simulink model "Inverter_block_for_test"  (R2022b)
settings: Solver=VariableStepAuto  StartTime=0.0  StopTime=10.0  RelTol=1e-3
libraries: rtican x2
settings Model: Creator=tiszu  LastModifiedBy=tiszu

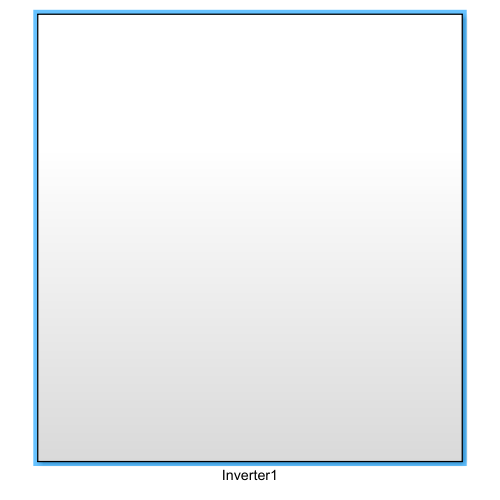
[thumbnail: Simulink's stored preview of the top-level diagram]
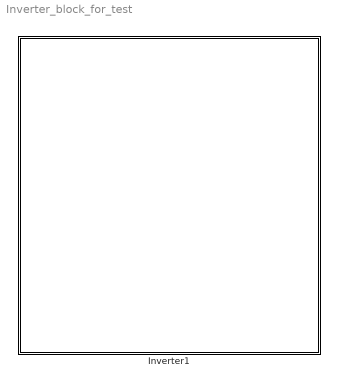
== system Inverter_block_for_test ==
  Inverter1 : Subsystem

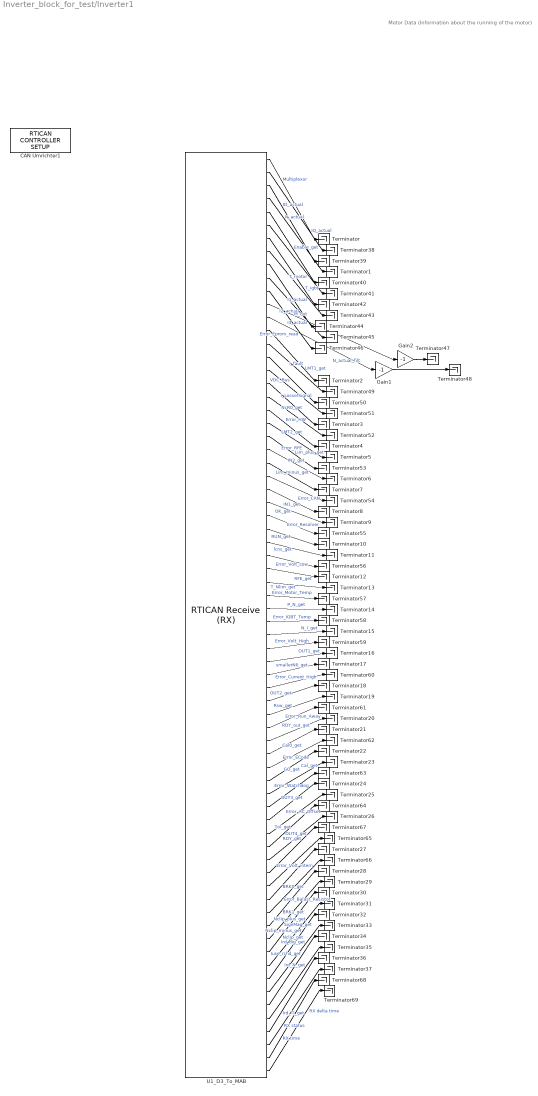
== system Inverter_block_for_test/Inverter1 ==
  note: Motor Data (Information about the running of the motor)
  CAN Umrichter1 : rtican/RTICAN CONTROLLER SETUP   Reserved1=[]  Reserved2=[]  Reserved3=[]  Reserved4=[]  AcceptanceMask=[]  ArbitrationField=[]  Parameters=[]  SFcnRTICANSettings=[]  MS_Struct=[]  BoardTypeNo=[]  BoardNo=[]  ChannelNo=[]  DialogFcn=[]  UnitName=[]  Revision=[]  UnitValues=[]  DSProperties=struct('RTI',struct('Version',uint32(12),'BlockType',struct('isSLSource',uint8(0),'isSLSink',uint8(0),'isHWSource',uint8(0),'isHWSink',uint8(0),'isSetup',uint8(1),'isInline',uint8(1),'isNonInline',uint8(0),'isInterrupt',uint8(0),'isChannelwise',uint8(0)),'IOBoardType','RTICAN','UnitType','NON_MESSAGE','Identifier','MASTER','DialogType','ML','BlockSet','RTICAN','SlaveProcessor','CAN'))  RTIBlockInterface=struct('InputPortsWidth',int32(0),'InputPortsActive',0,'OutputPortsWidth',int32(0),'OutputPortsActive',0,'DialogFcn','rtican_master_setup_gui','BlockDisplay',{{['CAN CONTROLLER\n SETUP'],'center'}},'IconTransparency','on','InitLevel',3,'IWork',{{{'',uint32(2)}}},'BlockName',struct('Token',{{'CAN_TYPE','_SETUP_M','_C'}},'BlockParam',{{'BoardTypeNo','BoardNo','ChannelNo'}}),'ParameterTunableNames',{{}})  RTIBlockParameters="struct('BoardTypeNo',{{1,'OFF',[]}},'BoardNo',{{2,'ON',[1 16]}},'ChannelNo',{{1,'ON',[1 2]}},'AcceptanceMask',{{0,'OFF',[]}},'ArbitrationField',{{0,'OFF',[]}},'Parameters',{{struct('Config',struct('Baudrate',1000,'SampleMode',1,'UsedParamSet',1,'validSettings',1,'isBTRvalues',0,'Advanced',struct('Baudrate',{500,500,500},'Frequency',{24000000,36000000,64000000},'Settings',{struct('SMPL',0,'BRP',0,'NBT',24,'TSEG1',15,'TSEG2',6,'SJW',3,'SP',70),struct('SMPL',0,'BRP',1,'NBT',18,'TSEG1',14,'TSEG2',1,'SJW',1,'SP',88),struct('SMPL',0,'BRP',3,'NBT',16,'TSEG1',12,'TSEG2',1,'SJW',1,'SP',87)},'BTR0',{192,65,67},'BTR1',{111,30,28})),'configType',1,'Options',struct('DataFileSelected',1,'DataFileName',{{'unitekinverter.dbc'}},'DataFileDate',{{['20-Jun-2024 23:32:37']}},'InterfaceFcn','rtican_dbc_file_parser','InterfaceFcnFileName','','LabelConfigType','volatile','AcceptanceMaskSelected',0,'MsgDataType','AllwaysDouble','NumType','hex','MaskType','STD','AcceptanceMask',0,'ArbitrationField',0,'UseMultipleMessageAccess',1),'RxReceiveStdOptions',struct('RxServiceStdEnabled',0,'RxServiceStdMsgIdent',1000,'RxServiceStdIdentNumType',1,'RxServiceStdIdentMask',0,'RxServiceStdMaskNumType',1,'RxServiceStdQueueSize',64),'RxReceiveXtdOptions',struct('RxServiceXtdEnabled',0,'RxServiceXtdMsgIdent',1001,'RxServiceXtdIdentNumType',1,'RxServiceXtdIdentMask',0,'RxServiceXtdMaskNumType',1,'RxServiceXtdQueueSize',64),'PartialNetworkingOptions',struct('switchedon',0,'format',1,'idmask',['    XXXXX XXXXXXXX XXXXXXXX XXXXXXXX'],'idcode','0','idfilter','0','datamaskused',0,'datalength',1,'datamask','0x0000000000000000','partialnetworkenable',0),'general',struct('Termination_common',1,'Termination_C252',1,'BusConfigurationRegister',0,'Transceiver','ISO11898','isFromLib',0)),'OFF',[]}},'CCPParameters',{{struct('CRO',struct('Format','STD','NumFormat','hex','Id',1639),'DTO',struct('Format','STD','NumFormat','hex','Id',2017),'StationAdr',struct('NumFormat','hex','Value',57),'StationId',struct('Value',['dSPACE CCP Service']),'Enabled',0),'OFF',[]}},'XCPParameters',{{struct('MASTER',struct('Format','STD','NumFormat','hex','Id',256),'SLAVE',struct('Format','STD','NumFormat','hex','Id',510),'Enabled',0,'PIDTransmissionEnabled',0),'OFF',[]}},'GroupId',{{struct('Group',{{'RTICAN'}},'No',4,'Behavior',{{'EVER'}},'BlockType',{{'SOURCE'}},'NameChangeFlag',1),'OFF',[]}},'SFcnRTICANSettings',{{struct('Baudrate',1000,'configType',1,'AdvancedConfig',struct('Frequency',{},'BTR0',{},'BTR1',{}),'UsedParamSet',1,'STDMaskSelected','no','XTDMaskSelected','no','BoardType','DS1','BoardNo',2,'ControllerNo',1,'Transceiver','ISO11898','BusConfigRegister',0,'TerminationRes',120,'UseMultipleMessageAccess','yes','STDRXSrvcUsed','no','STDRXSrvcMsgId',1000,'STDRXSrvcMsgMask',0,'STDRXSrvcQueueSize',64,'XTDRXSrvcUsed','no','XTDRXSrvcMsgId',1001,'XTDRXSrvcQueueSize',64,'XTDRXSrvcMsgMask',0,'PN_IsPNTransciever',0,'PN_IsPNEnabled',0,'PN_MsgFormat',1,'PN_idcode',0,'PN_idmask',2047,'PN_datamaskused',0,'PN_datalength',0,'PN_datamask',['0xFF, 0xFF, 0xFF, 0xFF, 0xFF, 0xFF, 0xFF, 0xFF']),'OFF',[]}},'SFcnRTICCPSettings',{{struct('CRO',struct('Format','STD','NumFormat','hex','Id',1639),'DTO',struct('Format','STD','NumFormat','hex','Id',2017),'StationAdr',struct('NumFormat','hex','Value',57),'StationId',struct('Value',['dSPACE CCP Service']),'Enabled',0),'OFF',[]}},'SFcnRTIXCPSettings',{{struct('MASTER',struct('Format','STD','NumFormat','hex','Id',256),'SLAVE',struct('Format','STD','NumFormat','hex','Id',510),'Enabled',0,'PIDTransmissionEnabled',0),'OFF',[]}},'TLCFileName',{{'rtican_master_setup','OFF',[]}})"  RTISFcnParameters=struct('SFcnRTICANSettings','struct','SFcnRTICCPSettings','struct','SFcnRTIXCPSettings','struct','AcceptanceMask','int32','ArbitrationField','int32','TLCFileName','char')  RTIBlockParaDefault="struct('BoardTypeNo',4302,'BoardNo',1,'ChannelNo',1,'AcceptanceMask',0,'ArbitrationField',0,'Parameters',struct('Config',struct('Baudrate',500,'SampleMode',1,'UsedParamSet',1,'validSettings',1,'isBTRvalues',0,'Advanced',struct('Frequency',16000000,'BTR0',64,'BTR1',28,'Settings',struct('SMPL',0,'BRP',0,'NBT',16,'TSEG1',12,'TSEG2',1,'SJW',1,'SP',87))),'configType',1,'Options',struct('DataFileSelected',0,'DataFileName',{{['<no datafile support>']}},'DataFileDate',{{''}},'InterfaceFcn','rtican_dbc_file_parser','InterfaceFcnFileName','','LabelConfigType','volatile','AcceptanceMaskSelected',0,'MsgDataType','AllwaysDouble','NumType','hex','MaskType','STD','AcceptanceMask',0,'ArbitrationField',0,'UseMultipleMessageAccess',0),'RxReceiveStdOptions',struct('RxServiceStdEnabled',0,'RxServiceStdMsgIdent',1000,'RxServiceStdIdentNumType',1,'RxServiceStdIdentMask',0,'RxServiceStdMaskNumType',1,'RxServiceStdQueueSize',64),'RxReceiveXtdOptions',struct('RxServiceXtdEnabled',0,'RxServiceXtdMsgIdent',1001,'RxServiceXtdIdentNumType',1,'RxServiceXtdIdentMask',0,'RxServiceXtdMaskNumType',1,'RxServiceXtdQueueSize',64),'PartialNetworkingOptions',struct('switchedon',0,'format',1,'idmask',['    XXXXX XXXXXXXX XXXXXXXX XXXXXXXX'],'idcode','0','idfilter','0','datamaskused',0,'datalength',1,'datamask','0x0000000000000000','partialnetworkenable',0),'general',struct('Termination_common',1,'Termination_C252',1,'BusConfigurationRegister',0,'Transceiver','ISO11898','isFromLib',1)),'CCPParameters',struct('CRO',struct('Format','STD','NumFormat','hex','Id',1639),'DTO',struct('Format','STD','NumFormat','hex','Id',2017),'StationAdr',struct('NumFormat','hex','Value',57),'StationId',struct('Value',['dSPACE CCP Service']),'Enabled',0),'XCPParameters',struct('MASTER',struct('Format','STD','NumFormat','hex','Id',256),'SLAVE',struct('Format','STD','NumFormat','hex','Id',510),'Enabled',0,'PIDTransmissionEnabled',0),'GroupId',struct('Group',{{'RTICAN'}},'No',1,'Behavior',{{'EVER'}},'BlockType',{{'SOURCE'}},'NameChangeFlag',1),'SFcnRTICANSettings',struct('Baudrate',500,'configType',1,'AdvandedConfig',struct('Frequency',16000000,'BTR0','0x40','BTR1','0x1C'),'UsedParamSet',1,'STDMaskSelected','no','XTDMaskSelected','no','BoardType','DS4302','BoardNo',1,'ControllerNo',1,'Transceiver','ISO11898','BusConfigRegister',0,'TerminationRes',120,'UseMultipleMessageAccess','no','STDRXSrvcUsed','no','STDRXSrvcMsgId',1000,'STDRXSrvcMsgMask',0,'STDRXSrvcQueueSize',64,'XTDRXSrvcUsed','no','XTDRXSrvcMsgId',1001,'XTDRXSrvcQueueSize',64,'XTDRXSrvcMsgMask',0),'SFcnRTICCPSettings',struct('CRO',struct('Format','STD','NumFormat','hex','Id',1639),'DTO',struct('Format','STD','NumFormat','hex','Id',2017),'StationAdr',struct('NumFormat','hex','Value',57),'StationId',struct('Value',['dSPACE CCP Service']),'Enabled',0),'SFcnRTIXCPSettings',struct('MASTER',struct('Format','STD','NumFormat','hex','Id',256),'SLAVE',struct('Format','STD','NumFormat','hex','Id',510),'Enabled',0,'PIDTransmissionEnabled',0),'TLCFileName','rtican_master_setup')"
      settings: AttributesFormatString=Group Id: RTICAN4\n
  Gain1 : Gain  Gain=-1
  Gain2 : Gain  Gain=-1
  Terminator{,1..69} (70 alike) : Terminator
  U1_D3_To_MAB : rtican/RTICAN Receive (RX)   Reserved1=[]  Reserved2=[]  Reserved3=[]  Reserved4=[]  SfcnMessage=[]  Msg_Struct=[]  BoardTypeNo=[]  BoardNo=[]  ChannelNo=[]  Parameters=[]  DialogFcn=[]  UnitName=[]  Revision=[]  UnitValues=[]  DSProperties=struct('RTI',struct('Version',uint32(5),'BlockType',struct('isSLSource',uint8(1),'isSLSink',uint8(1),'isHWSource',uint8(0),'isHWSink',uint8(0),'isSetup',uint8(0),'isInline',uint8(1),'isNonInline',uint8(0),'isInterrupt',uint8(0),'isChannelwise',uint8(0)),'IOBoardType','RTICAN','UnitType','MESSAGE','Identifier','RX','DialogType','MSVC','BlockSet','RTICAN','SlaveProcessor','CAN'))  RTIBlockInterface=struct('OutputPortsWidth',int32([1 1 1 1 1 1 1 1 1 1 1 1 1 1 1 1 1 1 1 1 1 1 1 1 1 1 1 1 1 1 1 1 1 1 1 1 1 1 1 1 1 1 1 1 1 1 1 1 1 1 1 1 1 1 1 1 1 1 1 1 1 1 1 1 1 1 1 1 1 1]),'OutputPortsActive',ones(1,70),'OutputPortsName',{{'Multiplexor','IQ_actual','ID_actual','N_actual','Enable_get','T_motor','T_igbt','I1_actual','I2_actual','I3_actual','Error_Eprom_read','M_out','N_actual_filt','LMT1_get','I_fault','VDC_Bus','I_LossofSignal','NcR0_get','Error_HW','LMT2_get','Lim_plus_get','Error_RFE','IN2_get','Lim_minus_get','Error_CAN','IN1_get','OK_get','Error_Resolver','RUN_get','lcns_get','Error_Volt_Low','RFE_get','T_Nlim_get','Error_Motor_Temp','P_N_get','Error_IGBT_Temp','N_I_get','Error_Volt_High','OUT1_get','smallerN0_get','Error_Current_High','OUT2_get','Rsw_get','Error_Run_Away','RDY_out_get','Cal0_get','Error_ECode','GO_get','Cal_get','Error_Watchdog','OUT3_get','Tol_get','Error_AC_Offset','OUT4_get','RDY_get','Error_Volt_intern','BRK0_get','Error_Balast_Resistor','BRK1_get','SignMag_get','Nclip_get','Nclip_plus_get','Nclip_minus_get','Ird_dig_get','Iuse_rchd_get','Ird_N_get','Ird_TI_get',['RX status'],['RX time'],['RX delta time']}},'OutputPortsDataType',{{'SS_DOUBLE','SS_DOUBLE','SS_DOUBLE','SS_DOUBLE','SS_DOUBLE','SS_DOUBLE','SS_DOUBLE','SS_DOUBLE','SS_DOUBLE','SS_DOUBLE','SS_DOUBLE','SS_DOUBLE','SS_DOUBLE','SS_DOUBLE','SS_DOUBLE','SS_DOUBLE','SS_DOUBLE','SS_DOUBLE','SS_DOUBLE','SS_DOUBLE','SS_DOUBLE','SS_DOUBLE','SS_DOUBLE','SS_DOUBLE','SS_DOUBLE','SS_DOUBLE','SS_DOUBLE','SS_DOUBLE','SS_DOUBLE','SS_DOUBLE','SS_DOUBLE','SS_DOUBLE','SS_DOUBLE','SS_DOUBLE','SS_DOUBLE','SS_DOUBLE','SS_DOUBLE','SS_DOUBLE','SS_DOUBLE','SS_DOUBLE','SS_DOUBLE','SS_DOUBLE','SS_DOUBLE','SS_DOUBLE','SS_DOUBLE','SS_DOUBLE','SS_DOUBLE','SS_DOUBLE','SS_DOUBLE','SS_DOUBLE','SS_DOUBLE','SS_DOUBLE','SS_DOUBLE','SS_DOUBLE','SS_DOUBLE','SS_DOUBLE','SS_DOUBLE','SS_DOUBLE','SS_DOUBLE','SS_DOUBLE','SS_DOUBLE','SS_DOUBLE','SS_DOUBLE','SS_DOUBLE','SS_DOUBLE','SS_DOUBLE','SS_DOUBLE','SS_DOUBLE','SS_DOUBLE','SS_DOUBLE'}},'OutputPortsLabel',{{'Multiplexor','IQ_actual','ID_actual','N_actual','Enable_get','T_motor','T_igbt','I1_actual','I2_actual','I3_actual','Error_Eprom_read','M_out','N_actual_filt','LMT1_get','I_fault','VDC_Bus','I_LossofSignal','NcR0_get','Error_HW','LMT2_get','Lim_plus_get','Error_RFE','IN2_get','Lim_minus_get','Error_CAN','IN1_get','OK_get','Error_Resolver','RUN_get','lcns_get','Error_Volt_Low','RFE_get','T_Nlim_get','Error_Motor_Temp','P_N_get','Error_IGBT_Temp','N_I_get','Error_Volt_High','OUT1_get','smallerN0_get','Error_Current_High','OUT2_get','Rsw_get','Error_Run_Away','RDY_out_get','Cal0_get','Error_ECode','GO_get','Cal_get','Error_Watchdog','OUT3_get','Tol_get','Error_AC_Offset','OUT4_get','RDY_get','Error_Volt_intern','BRK0_get','Error_Balast_Resistor','BRK1_get','SignMag_get','Nclip_get','Nclip_plus_get','Nclip_minus_get','Ird_dig_get','Iuse_rchd_get','Ird_N_get','Ird_TI_get',['RX status'],['RX time'],['RX delta time']}},'OutputPortsLabelMode','ON','InputPortsWidth',int32(0),'InputPortsActive',0,'DialogFcn','rtican_message_interface_gui','BlockDisplay',{{'','center'}},'IconTransparency','on','ParameterTunableNames',{{}},'InitLevel',3,'BlockName',struct('Token',{{'U1_D3_To_MAB'}}),'SampleTime',{{-1}},'TriggerPort',{{'none'}},'EnablePort',{{'none'}})  RTIBlockParameters=struct('BoardTypeNo',{{1,'OFF',[]}},'BoardNo',{{2,'ON',[1 16]}},'ChannelNo',{{1,'ON',[1 2]}},'Parameters',{{struct('DataFileSupport',struct('DataFileSelectedMaster',1,'DataFileSelectedLocal',1,'DataFileName','z:\023_exxe23\41_software_matlab\mab_e-traxx\unitekinverter.dbc|','DataFileDate',{{{['20-Jun-2024 23:32:37']}}},'SelectedFile','unitekinverter.dbc','InterfaceFcn','rtican_dbc_file_parser'),'Options',struct('StatusSelected',1,'TimeSelected',1,'DeltaTimeSelected',1,'BytePortSelected',0,'MessageLengthSelected',0,'TriggerPort',struct('Selected',0,'TriggerType',0),'UserCoding',struct('Selected',0,'InterfaceFile','UserDecodingFile','FcnName','UserDecodeFcn','InportSelected',0,'InportWidth',1,'OutportSelected',0,'OutportWidth',1),'EnablePortSelected',0,'SignalOnPortnameSelected',1,'UseRXService',0),'Message',struct('MsgOnBlocknameSelected',1,'MsgName','U1_D3_To_MAB','MsgIdFormat',0,'MsgId',385,'MsgLength',4,'NumSignals',67,'SampleTime',-1,'Signal',struct('SgnName',{'Multiplexor','IQ_actual','ID_actual','N_actual','Enable_get','T_motor','T_igbt','I1_actual','I2_actual','I3_actual','Error_Eprom_read','M_out','N_actual_filt','LMT1_get','I_fault','VDC_Bus','I_LossofSignal','NcR0_get','Error_HW','LMT2_get','Lim_plus_get','Error_RFE','IN2_get','Lim_minus_get','Error_CAN','IN1_get','OK_get','Error_Resolver','RUN_get','lcns_get','Error_Volt_Low','RFE_get','T_Nlim_get','Error_Motor_Temp','P_N_get','Error_IGBT_Temp','N_I_get','Error_Volt_High','OUT1_get','smallerN0_get','Error_Current_High','OUT2_get','Rsw_get','Error_Run_Away','RDY_out_get','Cal0_get','Error_ECode','GO_get','Cal_get','Error_Watchdog','OUT3_get','Tol_get','Error_AC_Offset','OUT4_get','RDY_get','Error_Volt_intern','BRK0_get','Error_Balast_Resistor','BRK1_get','SignMag_get','Nclip_get','Nclip_plus_get','Nclip_minus_get','Ird_dig_get','Iuse_rchd_get','Ird_N_get','Ird_TI_get'},'SgnStartBit',{0,8,8,8,8,8,8,8,8,8,8,8,8,8,8,8,8,9,9,9,10,10,10,11,11,11,12,12,12,13,13,13,14,14,15,15,16,16,16,17,17,17,18,18,18,19,19,19,20,20,20,21,21,21,22,22,23,23,23,24,25,26,27,28,29,30,31},'SgnLength',{8,12,12,16,1,16,16,12,12,12,1,16,16,1,1,15,1,1,1,1,1,1,1,1,1,1,1,1,1,1,1,1,1,1,1,1,1,1,1,1,1,1,1,1,1,1,1,1,1,1,1,1,1,1,1,1,1,1,1,1,1,1,1,1,1,1,1},'SgnType',{1,2,2,2,2,2,2,2,2,2,2,2,2,2,2,2,2,2,2,2,2,2,2,2,2,2,2,2,2,2,2,2,2,2,2,2,2,2,2,2,2,2,2,2,2,2,2,2,2,2,2,2,2,2,2,2,2,2,2,2,2,2,2,2,2,2,2},'ModeValue',{-1,39,40,48,64,73,74,84,85,86,143,160,168,216,233,235,236,64,143,216,64,143,216,64,143,216,64,143,216,64,143,216,64,143,64,143,64,143,216,64,143,216,64,143,216,64,143,216,64,143,216,64,143,216,64,143,64,143,216,64,64,64,64,64,64,64,64},'DataType',{0,1,1,1,0,0,1,1,1,1,1,1,1,0,0,0,0,0,1,0,0,1,0,0,1,0,0,1,0,0,1,0,0,1,0,1,0,1,0,0,1,0,0,1,0,0,1,0,0,1,0,0,1,0,0,1,0,1,0,0,0,0,0,0,0,0,0},'ByteLayout',{0,0,0,0,0,0,0,0,0,0,0,0,0,0,0,0,0,0,0,0,0,0,0,0,0,0,0,0,0,0,0,0,0,0,0,0,0,0,0,0,0,0,0,0,0,0,0,0,0,0,0,0,0,0,0,0,0,0,0,0,0,0,0,0,0,0,0},'Factor',{1,1,1,0.2288888,1,1,1,1,1,1,1,0.00440077,0.2288888,1,1,0.03166131439,1,1,1,1,1,1,1,1,1,1,1,1,1,1,1,1,1,1,1,1,1,1,1,1,1,1,1,1,1,1,1,1,1,1,1,1,1,1,1,1,1,1,1,1,1,1,1,1,1,1,1},'Offset',{0,0,0,0,0,0,0,0,0,0,0,0,0,0,0,0,0,0,0,0,0,0,0,0,0,0,0,0,0,0,0,0,0,0,0,0,0,0,0,0,0,0,0,0,0,0,0,0,0,0,0,0,0,0,0,0,0,0,0,0,0,0,0,0,0,0,0},'SgnComment',{{['Multiplexo for REGID']},{['Iq Quiescent current']},{['Direct winding current']},{['Speed value for Testing and calibration']},{['Get Enable status']},{['Temparatur of the Motor']},{['Temperature of the IGBT modules']},{['Motor Current Value for Phase 1']},{['Motor Current Value for Phase 2']},{['Motor Current Value for Phase 3']},{''},{['Torque Output value']},{['Speed value to be displayed']},{['Digital Input Limit 1']},{['Returns Faults from the Leistungsteil oder Power unit']},{['OverVoltage faults (only in Servo with Vdc-Bus messaging)']},{['Hardware Resolver Signal lost ']},{['Get Status of revolution lock (rev=0)']},{''},{['Digital Input Limit 2']},{['Get Status of positive Limitation']},{''},{['Digital Input Din 2']},{['Get Status of negative Limitation']},{''},{['Digital Input Din 1']},{['Get Status of drivetrain']},{''},{['Digital Input of software rotational field unlock RUN']},{['Get Status if current is limited to continous-current']},{''},{['Digital Input of hardware rotational field unlock RUN']},{['Get Status of torquelimited torque-mode']},{''},{['Get Status of positional control possible']},{''},{['Get status if revolution control is active']},{''},{['Digital Output Limit 1']},{['Get status if revolution is lower than 0.1% (standstill)']},{''},{['Digital Output Limit 2']},{['Get status if reference input is selected']},{''},{['Hardware relais-output BTB-Rdy']},{['Get Status if reference run is active']},{''},{['Status of internal unlock GO']},{['Get Status if reference position was recognized']},{''},{['Digital Output Limit 3']},{['Get Status if position is within the tolerance-window']},{''},{['Digital Output Limit 4']},{['Get Status if Inverter/Motor is ready to go']},{''},{['Get Status if non-excited brake on motor active']},{''},{['Status of the excited brake']},{['Get Status if target value is inverted']},{['Get Status in revolution limit is active (N_lim < 90%)']},{['Get Status if positive revolution limit via switch is active']},{['Get Status if negative revolution limit via switch is active']},{['Get Status if current limitation via switch is active']},{['Get Status if limit of current reduction is reached']},{['Get Status if current reduction via revolutions is active']},{['Get Status if current reduction via IGBT-Temperature is active']}},'SgnUnit',{'','','','','','','','','','','','','','','','','','','','','','','','','','','','','','','','','','','','','','','','','','','','','','','','','','','','','','','','','','','','','','','','','','',''},'Min',{0,-32768,-32768,-32768,0,-32767,-32768,-2048,-2048,-2048,0,-32768,-32768,0,0,0,0,0,0,0,0,0,0,0,0,0,0,0,0,0,0,0,0,0,0,0,0,0,0,0,0,0,0,0,0,0,0,0,0,0,0,0,0,0,0,0,0,0,0,0,0,0,0,0,0,0,0},'Max',{0,32767,32767,32767,0,32767,32767,2047,2047,2047,0,32767,32767,0,0,32767,0,0,0,0,0,0,1,0,0,1,0,0,1,0,0,1,0,0,0,0,0,0,0,0,0,0,0,0,0,0,0,0,0,0,0,0,0,0,0,0,0,0,0,0,0,0,0,0,0,0,0},'SLDataType',{'SS_DOUBLE','SS_DOUBLE','SS_DOUBLE','SS_DOUBLE','SS_DOUBLE','SS_DOUBLE','SS_DOUBLE','SS_DOUBLE','SS_DOUBLE','SS_DOUBLE','SS_DOUBLE','SS_DOUBLE','SS_DOUBLE','SS_DOUBLE','SS_DOUBLE','SS_DOUBLE','SS_DOUBLE','SS_DOUBLE','SS_DOUBLE','SS_DOUBLE','SS_DOUBLE','SS_DOUBLE','SS_DOUBLE','SS_DOUBLE','SS_DOUBLE','SS_DOUBLE','SS_DOUBLE','SS_DOUBLE','SS_DOUBLE','SS_DOUBLE','SS_DOUBLE','SS_DOUBLE','SS_DOUBLE','SS_DOUBLE','SS_DOUBLE','SS_DOUBLE','SS_DOUBLE','SS_DOUBLE','SS_DOUBLE','SS_DOUBLE','SS_DOUBLE','SS_DOUBLE','SS_DOUBLE','SS_DOUBLE','SS_DOUBLE','SS_DOUBLE','SS_DOUBLE','SS_DOUBLE','SS_DOUBLE','SS_DOUBLE','SS_DOUBLE','SS_DOUBLE','SS_DOUBLE','SS_DOUBLE','SS_DOUBLE','SS_DOUBLE','SS_DOUBLE','SS_DOUBLE','SS_DOUBLE','SS_DOUBLE','SS_DOUBLE','SS_DOUBLE','SS_DOUBLE','SS_DOUBLE','SS_DOUBLE','SS_DOUBLE','SS_DOUBLE'}),'MsgIdNumFormat',1,'MsgComment',{{''}}),'Version',1.2,'general',struct('isFromLib',0)),'OFF',[]}},'GroupId',{{struct('Group',{{'RTICAN'}},'No',4,'Behavior',{{'NAMECHANGE'}},'BlockType',{{'SINK'}},'NameChangeFlag',0),'OFF',[]}},'SFcnRTICANMessage',{{struct('MsgType','RX','SFcnPortType','Scalar','MsgName','U1_D3_To_MAB','MsgIdFormat','STD','MsgId',385,'MsgLength',4,'NumSignals',67,'SampleTime',-1,'Signal',struct('SgnName',{'Multiplexor','IQ_actual','ID_actual','N_actual','Enable_get','T_motor','T_igbt','I1_actual','I2_actual','I3_actual','Error_Eprom_read','M_out','N_actual_filt','LMT1_get','I_fault','VDC_Bus','I_LossofSignal','NcR0_get','Error_HW','LMT2_get','Lim_plus_get','Error_RFE','IN2_get','Lim_minus_get','Error_CAN','IN1_get','OK_get','Error_Resolver','RUN_get','lcns_get','Error_Volt_Low','RFE_get','T_Nlim_get','Error_Motor_Temp','P_N_get','Error_IGBT_Temp','N_I_get','Error_Volt_High','OUT1_get','smallerN0_get','Error_Current_High','OUT2_get','Rsw_get','Error_Run_Away','RDY_out_get','Cal0_get','Error_ECode','GO_get','Cal_get','Error_Watchdog','OUT3_get','Tol_get','Error_AC_Offset','OUT4_get','RDY_get','Error_Volt_intern','BRK0_get','Error_Balast_Resistor','BRK1_get','SignMag_get','Nclip_get','Nclip_plus_get','Nclip_minus_get','Ird_dig_get','Iuse_rchd_get','Ird_N_get','Ird_TI_get'},'SgnStartBit',{0,8,8,8,8,8,8,8,8,8,8,8,8,8,8,8,8,9,9,9,10,10,10,11,11,11,12,12,12,13,13,13,14,14,15,15,16,16,16,17,17,17,18,18,18,19,19,19,20,20,20,21,21,21,22,22,23,23,23,24,25,26,27,28,29,30,31},'SgnLength',{8,12,12,16,1,16,16,12,12,12,1,16,16,1,1,15,1,1,1,1,1,1,1,1,1,1,1,1,1,1,1,1,1,1,1,1,1,1,1,1,1,1,1,1,1,1,1,1,1,1,1,1,1,1,1,1,1,1,1,1,1,1,1,1,1,1,1},'SgnType',{'mode','mode-dependent','mode-dependent','mode-dependent','mode-dependent','mode-dependent','mode-dependent','mode-dependent','mode-dependent','mode-dependent','mode-dependent','mode-dependent','mode-dependent','mode-dependent','mode-dependent','mode-dependent','mode-dependent','mode-dependent','mode-dependent','mode-dependent','mode-dependent','mode-dependent','mode-dependent','mode-dependent','mode-dependent','mode-dependent','mode-dependent','mode-dependent','mode-dependent','mode-dependent','mode-dependent','mode-dependent','mode-dependent','mode-dependent','mode-dependent','mode-dependent','mode-dependent','mode-dependent','mode-dependent','mode-dependent','mode-dependent','mode-dependent','mode-dependent','mode-dependent','mode-dependent','mode-dependent','mode-dependent','mode-dependent','mode-dependent','mode-dependent','mode-dependent','mode-dependent','mode-dependent','mode-dependent','mode-dependent','mode-dependent','mode-dependent','mode-dependent','mode-dependent','mode-dependent','mode-dependent','mode-dependent','mode-dependent','mode-dependent','mode-dependent','mode-dependent','mode-dependent'},'ModeValue',{-1,39,40,48,64,73,74,84,85,86,143,160,168,216,233,235,236,64,143,216,64,143,216,64,143,216,64,143,216,64,143,216,64,143,64,143,64,143,216,64,143,216,64,143,216,64,143,216,64,143,216,64,143,216,64,143,64,143,216,64,64,64,64,64,64,64,64},'DataType',{['unsigned int'],['signed int'],['signed int'],['signed int'],['unsigned int'],['unsigned int'],['signed int'],['signed int'],['signed int'],['signed int'],['signed int'],['signed int'],['signed int'],['unsigned int'],['unsigned int'],['unsigned int'],['unsigned int'],['unsigned int'],['signed int'],['unsigned int'],['unsigned int'],['signed int'],['unsigned int'],['unsigned int'],['signed int'],['unsigned int'],['unsigned int'],['signed int'],['unsigned int'],['unsigned int'],['signed int'],['unsigned int'],['unsigned int'],['signed int'],['unsigned int'],['signed int'],['unsigned int'],['signed int'],['unsigned int'],['unsigned int'],['signed int'],['unsigned int'],['unsigned int'],['signed int'],['unsigned int'],['unsigned int'],['signed int'],['unsigned int'],['unsigned int'],['signed int'],['unsigned int'],['unsigned int'],['signed int'],['unsigned int'],['unsigned int'],['signed int'],['unsigned int'],['signed int'],['unsigned int'],['unsigned int'],['unsigned int'],['unsigned int'],['unsigned int'],['unsigned int'],['unsigned int'],['unsigned int'],['unsigned int']},'ByteLayout',{['little endian'],['little endian'],['little endian'],['little endian'],['little endian'],['little endian'],['little endian'],['little endian'],['little endian'],['little endian'],['little endian'],['little endian'],['little endian'],['little endian'],['little endian'],['little endian'],['little endian'],['little endian'],['little endian'],['little endian'],['little endian'],['little endian'],['little endian'],['little endian'],['little endian'],['little endian'],['little endian'],['little endian'],['little endian'],['little endian'],['little endian'],['little endian'],['little endian'],['little endian'],['little endian'],['little endian'],['little endian'],['little endian'],['little endian'],['little endian'],['little endian'],['little endian'],['little endian'],['little endian'],['little endian'],['little endian'],['little endian'],['little endian'],['little endian'],['little endian'],['little endian'],['little endian'],['little endian'],['little endian'],['little endian'],['little endian'],['little endian'],['little endian'],['little endian'],['little endian'],['little endian'],['little endian'],['little endian'],['little endian'],['little endian'],['little endian'],['little endian']},'Factor',{1,1,1,0.2288888,1,1,1,1,1,1,1,0.00440077,0.2288888,1,1,0.03166131439,1,1,1,1,1,1,1,1,1,1,1,1,1,1,1,1,1,1,1,1,1,1,1,1,1,1,1,1,1,1,1,1,1,1,1,1,1,1,1,1,1,1,1,1,1,1,1,1,1,1,1},'Offset',{0,0,0,0,0,0,0,0,0,0,0,0,0,0,0,0,0,0,0,0,0,0,0,0,0,0,0,0,0,0,0,0,0,0,0,0,0,0,0,0,0,0,0,0,0,0,0,0,0,0,0,0,0,0,0,0,0,0,0,0,0,0,0,0,0,0,0},'SLDataType',{'SS_DOUBLE','SS_DOUBLE','SS_DOUBLE','SS_DOUBLE','SS_DOUBLE','SS_DOUBLE','SS_DOUBLE','SS_DOUBLE','SS_DOUBLE','SS_DOUBLE','SS_DOUBLE','SS_DOUBLE','SS_DOUBLE','SS_DOUBLE','SS_DOUBLE','SS_DOUBLE','SS_DOUBLE','SS_DOUBLE','SS_DOUBLE','SS_DOUBLE','SS_DOUBLE','SS_DOUBLE','SS_DOUBLE','SS_DOUBLE','SS_DOUBLE','SS_DOUBLE','SS_DOUBLE','SS_DOUBLE','SS_DOUBLE','SS_DOUBLE','SS_DOUBLE','SS_DOUBLE','SS_DOUBLE','SS_DOUBLE','SS_DOUBLE','SS_DOUBLE','SS_DOUBLE','SS_DOUBLE','SS_DOUBLE','SS_DOUBLE','SS_DOUBLE','SS_DOUBLE','SS_DOUBLE','SS_DOUBLE','SS_DOUBLE','SS_DOUBLE','SS_DOUBLE','SS_DOUBLE','SS_DOUBLE','SS_DOUBLE','SS_DOUBLE','SS_DOUBLE','SS_DOUBLE','SS_DOUBLE','SS_DOUBLE','SS_DOUBLE','SS_DOUBLE','SS_DOUBLE','SS_DOUBLE','SS_DOUBLE','SS_DOUBLE','SS_DOUBLE','SS_DOUBLE','SS_DOUBLE','SS_DOUBLE','SS_DOUBLE','SS_DOUBLE'}),'StatusSelected','yes','TimeSelected','yes','DeltaTimeSelected','yes','BytePortSelected','no','MessageLengthSelected','no','TriggerPort',struct('Selected','no','TriggerType',0),'UserCoding',struct('Selected','no','InterfaceFile','UserDecodingFile','FcnName','UserDecodeFcn','InportSelected','no','InportWidth',1,'OutportSelected','no','OutportWidth',1),'EnablePortSelected','no','UseRXService','no','BoardType','DS1','BoardNo',2,'ControllerNo',1),'OFF',[]}},'TLCFileName',{{'rtican_rx_message','OFF',[]}})  RTISFcnParameters=struct('SFcnRTICANMessage','struct','TLCFileName','char')  RTIBlockParaDefault=struct('BoardTypeNo',4302,'BoardNo',1,'ChannelNo',1,'Parameters',struct('DataFileSupport',struct('DataFileSelectedMaster',0,'DataFileSelectedLocal',0,'DataFileName','','DataFileDate','','SelectedFile',['<no file selected>']),'Options',struct('StatusSelected',1,'TimeSelected',1,'DeltaTimeSelected',1,'BytePortSelected',0,'MessageLengthSelected',0,'TriggerPort',struct('Selected',0,'TriggerType','rising'),'UserCoding',struct('Selected',0,'InterfaceFile','UserDecodingFile','FcnName','UserDecodeFcn','InportSelected',0,'InportWidth',1,'OutportSelected',0,'OutportWidth',1),'EnablePortSelected',0,'SignalOnPortnameSelected',1,'UseRXService',0),'Message',struct('MsgOnBlocknameSelected',0,'MsgName',['RX Message'],'MsgIdFormat',0,'MsgId',100,'MsgLength',8,'NumSignals',1,'SampleTime',-1,'Signal',struct('SgnName',['RX signal'],'SgnStartBit',0,'SgnLength',8,'SgnType',0,'ModeValue',-1,'DataType',0,'SLDataType','SS_DOUBLE','ByteLayout',0,'Factor',1,'Offset',0,'Min',0,'Max',255,'SgnComment',{{}},'SgnUnit',''),'MsgIdNumFormat',0,'MsgComment',{{''}}),'Version',1.2,'general',struct('isFromLib',1)),'GroupId',struct('Group',{{'RTICAN'}},'No',1,'Behavior',{{'NAMECHANGE'}},'BlockType',{{'SINK'}},'NameChangeFlag',0),'SFcnRTICANMessage',struct('MsgType','RX','MsgName',['RX Message'],'MsgIdFormat','STD','MsgId',100,'MsgLength',8,'NumSignals',1,'SampleTime',-1,'Signal',struct('SgnName',['RX signal'],'SgnStartBit',0,'SgnLength',8,'SgnType','standard','ModeValue',-1,'DataType',['unsigned int'],'ByteLayout',['little endian'],'SLDataType','SS_DOUBLE','Factor',1,'Offset',0),'StatusSelected','yes','TimeSelected','yes','DeltaTimeSelected','yes','BytePortSelected','no','MessageLengthSelected','no','EnablePortSelected','no','UserCoding',struct('Selected','no','InterfaceFile','UserDecodingFile','FcnName','UserDecodeFcn','InportSelected','no','InportWidth',1,'OutportSelected','no','OutportWidth',1),'TriggerPort',struct('Selected','no','TriggerType','rising'),'UseRXService','no','BoardType','DS4302','BoardNo',1,'ControllerNo',1,'SFcnPortType','Scalar'),'TLCFileName','rtican_rx_message')
      settings: AttributesFormatString=Group Id: RTICAN4\n
  wires:
  U1_D3_To_MAB/70 -> Terminator69/1  "RX delta time"
  U1_D3_To_MAB/69 -> Terminator68/1  "RX time"
  U1_D3_To_MAB/5 -> Terminator40/1  "Enable_get"
  U1_D3_To_MAB/55 -> Terminator67/1  "RDY_get"
  U1_D3_To_MAB/8 -> Terminator43/1  "I1_actual"
  U1_D3_To_MAB/9 -> Terminator44/1  "I2_actual"
  U1_D3_To_MAB/10 -> Terminator45/1  "I3_actual"
  U1_D3_To_MAB/2 -> Terminator38/1  "IQ_actual"
  U1_D3_To_MAB/3 -> Terminator39/1  "ID_actual"
  U1_D3_To_MAB/13 -> Gain1/1  "N_actual_filt"
  U1_D3_To_MAB/6 -> Terminator41/1  "T_motor"
  U1_D3_To_MAB/7 -> Terminator42/1  "T_igbt"
  U1_D3_To_MAB/12 -> Gain2/1  "M_out"
  U1_D3_To_MAB/15 -> Terminator49/1  "I_fault"
  U1_D3_To_MAB/17 -> Terminator51/1  "I_LossofSignal"
  U1_D3_To_MAB/16 -> Terminator50/1  "VDC_Bus"
  U1_D3_To_MAB/50 -> Terminator63/1  "Error_Watchdog"
  U1_D3_To_MAB/34 -> Terminator57/1  "Error_Motor_Temp"
  U1_D3_To_MAB/28 -> Terminator55/1  "Error_Resolver"
  U1_D3_To_MAB/56 -> Terminator65/1  "Error_Volt_intern"
  U1_D3_To_MAB/25 -> Terminator54/1  "Error_CAN"
  U1_D3_To_MAB/19 -> Terminator52/1  "Error_HW"
  U1_D3_To_MAB/53 -> Terminator64/1  "Error_AC_Offset"
  U1_D3_To_MAB/36 -> Terminator58/1  "Error_IGBT_Temp"
  U1_D3_To_MAB/47 -> Terminator62/1  "Error_ECode"
  U1_D3_To_MAB/44 -> Terminator61/1  "Error_Run_Away"
  U1_D3_To_MAB/38 -> Terminator59/1  "Error_Volt_High"
  U1_D3_To_MAB/41 -> Terminator60/1  "Error_Current_High"
  U1_D3_To_MAB/31 -> Terminator56/1  "Error_Volt_Low"
  U1_D3_To_MAB/58 -> Terminator66/1  "Error_Balast_Resistor"
  U1_D3_To_MAB/22 -> Terminator53/1  "Error_RFE"
  U1_D3_To_MAB/11 -> Terminator46/1  "Error_Eprom_read"
  Gain1/1 -> Terminator48/1
  Gain2/1 -> Terminator47/1
  U1_D3_To_MAB/1 -> Terminator/1  "Multiplexor"
  U1_D3_To_MAB/4 -> Terminator1/1  "N_actual"
  U1_D3_To_MAB/14 -> Terminator2/1  "LMT1_get"
  U1_D3_To_MAB/18 -> Terminator3/1  "NcR0_get"
  U1_D3_To_MAB/20 -> Terminator4/1  "LMT2_get"
  U1_D3_To_MAB/21 -> Terminator5/1  "Lim_plus_get"
  U1_D3_To_MAB/23 -> Terminator6/1  "IN2_get"
  U1_D3_To_MAB/24 -> Terminator7/1  "Lim_minus_get"
  U1_D3_To_MAB/26 -> Terminator8/1  "IN1_get"
  U1_D3_To_MAB/27 -> Terminator9/1  "OK_get"
  U1_D3_To_MAB/29 -> Terminator10/1  "RUN_get"
  U1_D3_To_MAB/30 -> Terminator11/1  "lcns_get"
  U1_D3_To_MAB/32 -> Terminator12/1  "RFE_get"
  U1_D3_To_MAB/33 -> Terminator13/1  "T_Nlim_get"
  U1_D3_To_MAB/35 -> Terminator14/1  "P_N_get"
  U1_D3_To_MAB/37 -> Terminator15/1  "N_I_get"
  U1_D3_To_MAB/39 -> Terminator16/1  "OUT1_get"
  U1_D3_To_MAB/40 -> Terminator17/1  "smallerN0_get"
  U1_D3_To_MAB/42 -> Terminator18/1  "OUT2_get"
  U1_D3_To_MAB/43 -> Terminator19/1  "Rsw_get"
  U1_D3_To_MAB/45 -> Terminator20/1  "RDY_out_get"
  U1_D3_To_MAB/46 -> Terminator21/1  "Cal0_get"
  U1_D3_To_MAB/48 -> Terminator22/1  "GO_get"
  U1_D3_To_MAB/49 -> Terminator23/1  "Cal_get"
  U1_D3_To_MAB/51 -> Terminator24/1  "OUT3_get"
  U1_D3_To_MAB/52 -> Terminator25/1  "Tol_get"
  U1_D3_To_MAB/54 -> Terminator26/1  "OUT4_get"
  U1_D3_To_MAB/57 -> Terminator27/1  "BRK0_get"
  U1_D3_To_MAB/59 -> Terminator28/1  "BRK1_get"
  U1_D3_To_MAB/60 -> Terminator29/1  "SignMag_get"
  U1_D3_To_MAB/61 -> Terminator30/1  "Nclip_get"
  U1_D3_To_MAB/62 -> Terminator31/1  "Nclip_plus_get"
  U1_D3_To_MAB/63 -> Terminator32/1  "Nclip_minus_get"
  U1_D3_To_MAB/64 -> Terminator33/1  "Ird_dig_get"
  U1_D3_To_MAB/65 -> Terminator34/1  "Iuse_rchd_get"
  U1_D3_To_MAB/66 -> Terminator35/1  "Ird_N_get"
  U1_D3_To_MAB/67 -> Terminator36/1  "Ird_TI_get"
  U1_D3_To_MAB/68 -> Terminator37/1  "RX status"
